simulink model "servoSlorV2"  (R2022a)
settings: Solver=VariableStepAuto  StartTime=0.0  StopTime=30  RelTol=1e-3
undefined symbols (not defined in the file): sigbuilder_block
libraries: simulink x4
settings Model: Creator=User  LastModifiedBy=User

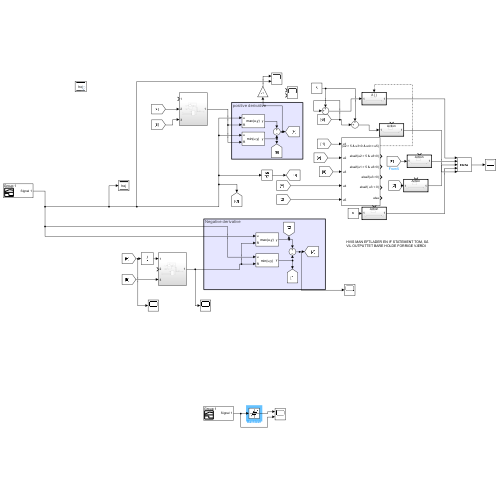
[thumbnail: Simulink's stored preview of the top-level diagram]
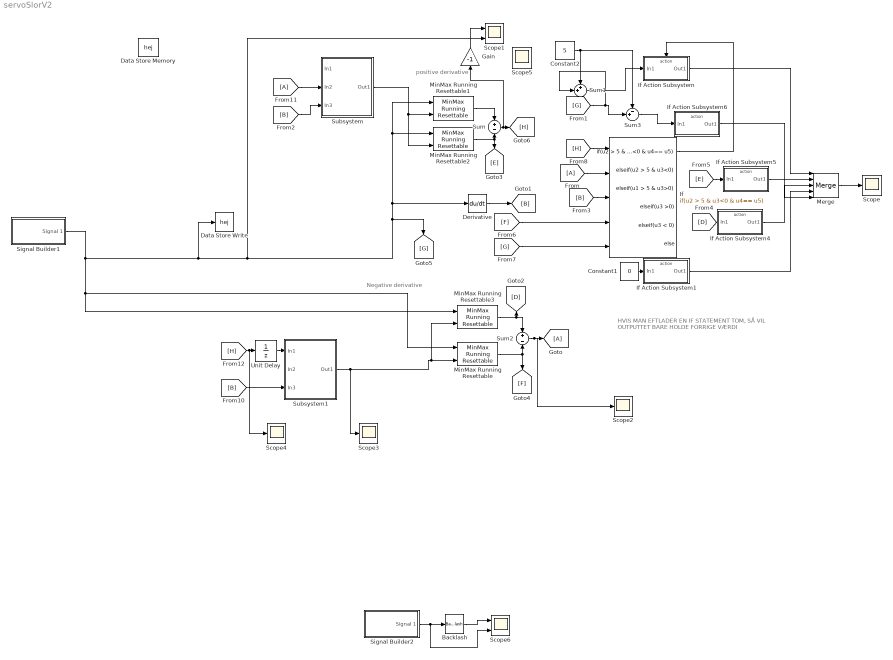
== system servoSlorV2 ==
  note: HVIS MAN EFTLADER EN IF STATEMENT TOM, SÅ VIL OUTPUTTET BARE HOLDE FORRIGE VÆRDI
  note: positive derivative
  note: Negative derivative
  Backlash : Backlash  BacklashWidth=5
  Constant1 : Constant  Value=0
  Constant2 : Constant  Value=5
  Data Store Memory : DataStoreMemory  DataStoreName=hej  WriteAfterWriteMsg=warning  ShowAdditionalParam=off  DataLoggingName=hej
      settings: DataLoggingNameMode=Custom
  Data Store Write : DataStoreWrite  DataStoreName=hej  IndexOptions=Index vector (dialog)  Indices=1  OutputSizes=1
  Derivative : Derivative
  From : From
  From11 : From
  Gain : Gain  Gain=-1
  Goto : Goto
  If : If  NumInputs=5  IfExpression=u2 > 5 & u3<0 & u4== u5  ElseIfExpressions=u2 > 5 & u3<0,u1 > 5 & u3>0,u3 >0, u3 < 0
  If Action Subsystem : Subsystem  TreatAsAtomicUnit=on
  If Action Subsystem1 : Subsystem  TreatAsAtomicUnit=on
  If Action Subsystem4 : Subsystem  TreatAsAtomicUnit=on
  If Action Subsystem5 : Subsystem  TreatAsAtomicUnit=on
  If Action Subsystem6 : Subsystem  TreatAsAtomicUnit=on
  Merge : Merge  Inputs=5
  MinMax Running Resettable : simulink/Math Operations/MinMax Running Resettable  Function=min  vinit=0.0
  MinMax Running Resettable1 : simulink/Math Operations/MinMax Running Resettable  Function=max  vinit=0.0
  MinMax Running Resettable2 : simulink/Math Operations/MinMax Running Resettable  Function=min  vinit=0
  MinMax Running Resettable3 : simulink/Math Operations/MinMax Running Resettable  Function=max  vinit=0.0
  Scope{,2..4} (4 alike) : Scope
  Scope1 : Scope  NumInputPorts=2
  Scope5 : Scope  NumInputPorts=2
  Scope6 : Scope  NumInputPorts=2
  Signal Builder1 : Subsystem  Tag=STV Subsys  LoadFcn=sigbuilder_block('load',[76.5 207 448.5 239 ]);  StartFcn=sigbuilder_block('start');  StopFcn=sigbuilder_block('stop');  ClipboardFcn=sigbuilder_block('clipboard');  mask(Sigbuilder block){tuvar=[0:10]}
      mask help: Simulink:masks:SigbuilderBlock_MD
      mask init:
      | if ~strcmp(get_param(bdroot(gcbh),'SimulationStatus'),'stopped') tuvar = sigbuilder_block('maskInit'); end
      settings: CopyFcn=sigbuilder_block('copy');  DeleteFcn=sigbuilder_block('delete');  ModelCloseFcn=sigbuilder_block('modelClose');  PreSaveFcn=sigbuilder_block('preSave');  PauseFcn=sigbuilder_block('pause');  ContinueFcn=sigbuilder_block('continue');  NameChangeFcn=sigbuilder_block('namechange');  OpenFcn=sigbuilder_block('open',[76.5 207 448.5 239 ]);  CloseFcn=sigbuilder_block('close');
      mask Display: plot(0, 0, 100, 100,[2, 2, 32, 32, 2], [68, 8, 8, 68, 68],[32, 2], [38, 38], [32, 19, 2],[53, 60, 44], [32, 17, 17, 2],[16, 16, 31, 31]);txt = getActiveGroup(gcbh);text(2, 100, txt,'verticalAlignment', 'top');
  Signal Builder2 : Subsystem  Tag=STV Subsys  LoadFcn=sigbuilder_block('load');  StartFcn=sigbuilder_block('start');  StopFcn=sigbuilder_block('stop');  ClipboardFcn=sigbuilder_block('clipboard');  mask(Sigbuilder block){tuvar=[0:10]}
      mask help: Simulink:masks:SigbuilderBlock_MD
      mask init:
      | if ~strcmp(get_param(bdroot(gcbh),'SimulationStatus'),'stopped') tuvar = sigbuilder_block('maskInit'); end
      settings: CopyFcn=sigbuilder_block('copy');  DeleteFcn=sigbuilder_block('delete');  ModelCloseFcn=sigbuilder_block('modelClose');  PreSaveFcn=sigbuilder_block('preSave');  PauseFcn=sigbuilder_block('pause');  ContinueFcn=sigbuilder_block('continue');  NameChangeFcn=sigbuilder_block('namechange');  OpenFcn=sigbuilder_block('open',[76.5 207 448.5 239 ]);  CloseFcn=sigbuilder_block('close');
      mask Display: plot(0, 0, 100, 100,[2, 2, 32, 32, 2], [68, 8, 8, 68, 68],[32, 2], [38, 38], [32, 19, 2],[53, 60, 44], [32, 17, 17, 2],[16, 16, 31, 31]);txt = getActiveGroup(gcbh);text(2, 100, txt,'verticalAlignment', 'top');
  Subsystem : Subsystem
  Subsystem1 : Subsystem
  Sum : Sum  Inputs=+-
  Sum1 : Sum  Inputs=++|
  Sum2 : Sum  Inputs=+-
  Sum3 : Sum  Inputs=-+|
  Unit Delay : UnitDelay  SampleTime=0.001  HasFrameUpgradeWarning=on
  wires:
  If Action Subsystem/1(Out1) -> Merge/1
  Merge/1 -> Scope/1
  Sum1/1 -> If Action Subsystem/1(In1)
  Constant2/1 -> Sum3/1, Sum1/1
  MinMax Running Resettable3/1 -> [D], Sum2/1
  MinMax Running Resettable2/1 -> [E], Sum/2
  MinMax Running Resettable1/1 -> Sum/1
  If/1 -> If Action Subsystem/Action
  Sum2/1 -> Scope2/1, Goto/1
  From/1 -> If/2
  Constant1/1 -> If Action Subsystem1/1(In1)
  MinMax Running Resettable/1 -> [F], Sum2/2
  Signal Builder1/1(Signal 1) -> MinMax Running Resettable/1, MinMax Running Resettable3/1, Data Store Write/1, Scope1/2, MinMax Running Resettable1/1, MinMax Running Resettable2/1, Derivative/1, [G]
  Derivative/1 -> [B]
  [B] -> If/3
  [D] -> If Action Subsystem4/1(In1)
  [E] -> If Action Subsystem5/1(In1)
  If Action Subsystem5/1(Out1) -> Merge/2
  If Action Subsystem4/1(Out1) -> Merge/3
  If Action Subsystem1/1(Out1) -> Merge/4
  Sum3/1 -> If Action Subsystem6/1(In1)
  If Action Subsystem6/1(Out1) -> Merge/5
  [F] -> If/4
  [G] -> If/5
  [H] -> If/1
  [G] -> Sum1/2, Sum3/2
  Subsystem1/1(Out1) -> Scope3/1, MinMax Running Resettable3/2, MinMax Running Resettable/2
  Subsystem/1(Out1) -> MinMax Running Resettable2/2, MinMax Running Resettable1/2
  From11/1 -> Subsystem/2(In2)
  [B] -> Subsystem/3(In3)
  [B] -> Subsystem1/3(In3)
  Sum/1 -> Gain/1, [H]
  [H] -> Scope4/1, Unit Delay/1
  Unit Delay/1 -> Subsystem1/1(In1)
  Gain/1 -> Scope1/1
  Signal Builder2/1(Signal 1) -> Scope6/2, Backlash/1
  Backlash/1 -> Scope6/1

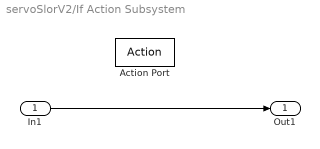
== system servoSlorV2/If Action Subsystem ==
  In1 : Inport
  Action Port : ActionPort  ActionPortLabel=if(u2 > 5 & u3<0 & u4== u5)
  Out1 : Outport
  wires:
  In1/1 -> Out1/1

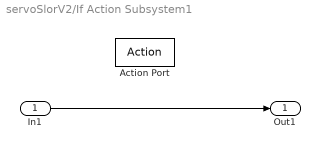
== system servoSlorV2/If Action Subsystem1 ==
  In1 : Inport
  Action Port : ActionPort
  Out1 : Outport
  wires:
  In1/1 -> Out1/1

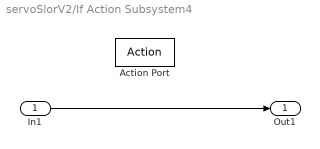
== system servoSlorV2/If Action Subsystem4 ==
  In1 : Inport
  Action Port : ActionPort
  Out1 : Outport
  wires:
  In1/1 -> Out1/1

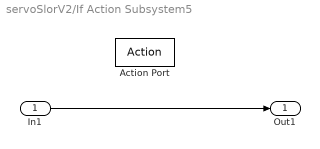
== system servoSlorV2/If Action Subsystem5 ==
  In1 : Inport
  Action Port : ActionPort
  Out1 : Outport
  wires:
  In1/1 -> Out1/1

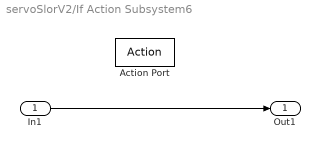
== system servoSlorV2/If Action Subsystem6 ==
  In1 : Inport
  Action Port : ActionPort
  Out1 : Outport
  wires:
  In1/1 -> Out1/1

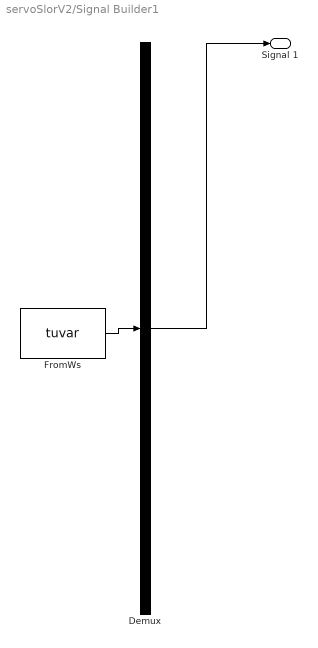
== system servoSlorV2/Signal Builder1 ==
  Demux : Demux  Tag=STV Demux  Outputs=1
      settings: DisplayOption=none
  FromWs : FromWorkspace  Tag=STV FromWs  VariableName=tuvar
      SigBuilderData=|
      | common.afterFinalStr = 'Extrapolate'
      | common.sampleTime = 0
      | dataSet.timeRange = [0 30]
      | dataSet.name = 'Group 1'
      | sbobj.Groups.Name = 'Group 1'
      | sbobj.Groups.Signals.Name = 'Signal 1'
      | sbobj.Groups.Signals.XData = [0 5 6 7 8.5 10 15 17.5 20 30]
      | sbobj.Groups.Signals.YData = [0 0 -15 -12 -25 0 0 20 0 0]
      | sbobj.Groups.TimeRange = [0 30]
  Signal 1 : Outport  Tag=STV Outport
  wires:
  Demux/1 -> Signal 1/1
  FromWs/1 -> Demux/1

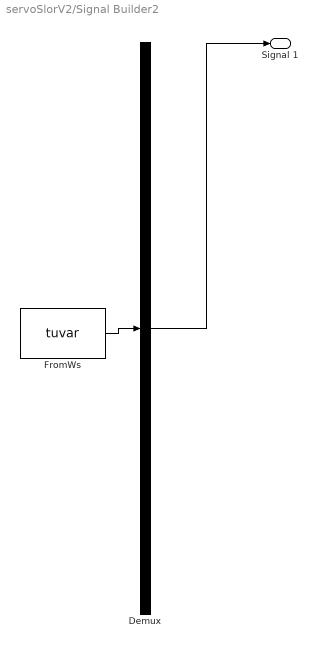
== system servoSlorV2/Signal Builder2 ==
  Demux : Demux  Tag=STV Demux  Outputs=1
      settings: DisplayOption=none
  FromWs : FromWorkspace  Tag=STV FromWs  VariableName=tuvar
      SigBuilderData=|
      | common.afterFinalStr = 'Extrapolate'
      | common.sampleTime = 0
      | dataSet.timeRange = [0 30]
      | dataSet.name = 'Group 1'
      | sbobj.Groups.Name = 'Group 1'
      | sbobj.Groups.Signals.Name = 'Signal 1'
      | sbobj.Groups.Signals.XData = [0 5 6 7 8.5 10 15 17.5 20 30]
      | sbobj.Groups.Signals.YData = [0 0 -15 -12 -25 0 0 20 0 0]
      | sbobj.Groups.TimeRange = [0 30]
  Signal 1 : Outport  Tag=STV Outport
  wires:
  Demux/1 -> Signal 1/1
  FromWs/1 -> Demux/1

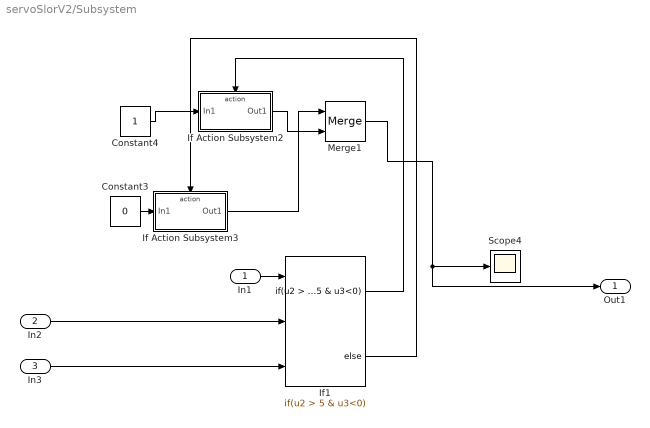
== system servoSlorV2/Subsystem ==
  In1 : Inport
  In2 : Inport  Port=2
  In3 : Inport  Port=3
  Constant3 : Constant  Value=0
  Constant4 : Constant
  If Action Subsystem2 : Subsystem  TreatAsAtomicUnit=on
  If Action Subsystem3 : Subsystem  TreatAsAtomicUnit=on
  If1 : If  NumInputs=3  IfExpression=u2 > 5 & u3<0
  Merge1 : Merge
  Scope4 : Scope
  Out1 : Outport
  wires:
  In3/1 -> If1/3
  If1/2 -> If Action Subsystem3/Action
  If Action Subsystem2/1(Out1) -> Merge1/2
  Constant4/1 -> If Action Subsystem2/1(In1)
  In2/1 -> If1/2
  Merge1/1 -> Out1/1, Scope4/1
  Constant3/1 -> If Action Subsystem3/1(In1)
  If Action Subsystem3/1(Out1) -> Merge1/1
  If1/1 -> If Action Subsystem2/Action
  In1/1 -> If1/1

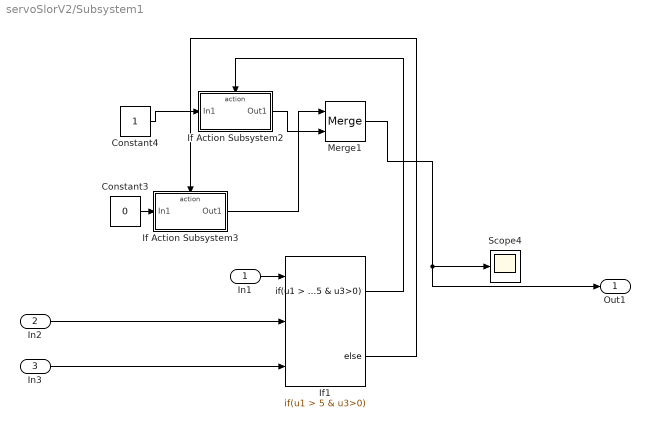
== system servoSlorV2/Subsystem1 ==
  In1 : Inport
  In2 : Inport  Port=2
  In3 : Inport  Port=3
  Constant3 : Constant  Value=0
  Constant4 : Constant
  If Action Subsystem2 : Subsystem  TreatAsAtomicUnit=on
  If Action Subsystem3 : Subsystem  TreatAsAtomicUnit=on
  If1 : If  NumInputs=3  IfExpression=u1 > 5 & u3>0
  Merge1 : Merge
  Scope4 : Scope
  Out1 : Outport
  wires:
  In3/1 -> If1/3
  If1/2 -> If Action Subsystem3/Action
  If Action Subsystem2/1(Out1) -> Merge1/2
  Constant4/1 -> If Action Subsystem2/1(In1)
  In2/1 -> If1/2
  Merge1/1 -> Out1/1, Scope4/1
  Constant3/1 -> If Action Subsystem3/1(In1)
  If Action Subsystem3/1(Out1) -> Merge1/1
  If1/1 -> If Action Subsystem2/Action
  In1/1 -> If1/1

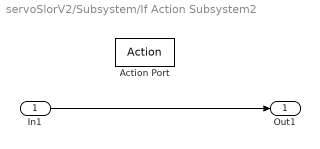
== system servoSlorV2/Subsystem/If Action Subsystem2 ==
  In1 : Inport
  Action Port : ActionPort  ActionPortLabel=if(u2 > 5 & u3<0)
  Out1 : Outport
  wires:
  In1/1 -> Out1/1

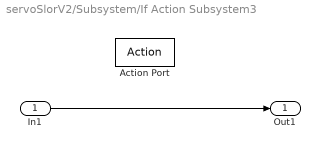
== system servoSlorV2/Subsystem/If Action Subsystem3 ==
  In1 : Inport
  Action Port : ActionPort  ActionPortLabel=else
  Out1 : Outport
  wires:
  In1/1 -> Out1/1

== system servoSlorV2/Subsystem1/If Action Subsystem2 ==
  In1 : Inport
  Action Port : ActionPort  ActionPortLabel=if(u1 > 5 & u3>0)
  Out1 : Outport
  wires:
  In1/1 -> Out1/1

== system servoSlorV2/Subsystem1/If Action Subsystem3 ==
  In1 : Inport
  Action Port : ActionPort  ActionPortLabel=else
  Out1 : Outport
  wires:
  In1/1 -> Out1/1
